simulink model "CRReferenceApplication"  (R2020a)
settings: Solver=ode23tb  StartTime=0.0  StopTime=60  FixedStep=.001  RelTol=1e-3  EnableMultiTasking=on
StartFcn:
  | %tic
StopFcn:
  | %toc
model workspace (MAT data in the model file):
  A_mu = 10
  B_reff = 8.386
  Cz = 7766.25
  DCT_Param.Transmission.Ratios = [3.78 2.18 1.43 1.03 0.935 0.84]
  DCT_Param.Transmission.Shaft_Inertia_Odd = 0.0023
  DCT_Param.Transmission.Shaft_Inertia_Even = 0.0009
  DCT_Param.Transmission.Shaft_Inertia_Output = 0.008
  DCT_Param.Transmission.Gear_Inertia = 0.001
  DCT_Param.Transmission.Gear_Efficiency = 0.94
  DCT_Param.Transmission.Gear_Ang_Vel_Thr = 0.01
  DCT_Param.Transmission.Shaft_Velocity_Odd = 0
  DCT_Param.Transmission.Shaft_Velocity_Even = 0
  DCT_Param.Transmission.Shaft_Velocity_Output = 0
  DCT_Param.Transmission.Gear_Initial_Velocity = 0
  DCT_Param.Transmission.Abstract.Compliance = 100000
  DCT_Param.Transmission.Abstract.Damping = 10000
  DCT_Param.Transmission.Abstract.Ratio_Time_Const = 0.05
  DCT_Param.Transmission.Abstract.Shift_Gear_Delay = 25
  DCT_Param.Clutch.Torque_Radius = 130
  DCT_Param.Clutch.Num_Friction_Surfaces = 4
  DCT_Param.Clutch.Engagement_Piston_Area = 0.001
  DCT_Param.Clutch.Kinetic_Friction_Coeff = 0.3
  DCT_Param.Clutch.Static_Friction_Coeff = 0.31
  DCT_Param.Clutch.Derating_Factor = 1
  DCT_Param.Clutch.Clutch_Velocity_Tolerance = 0.001
  DCT_Param.Clutch.Threshold_Pressure = 1
  DCT_Param.Clutch.Drag_Torque_Coeff = 0
  DCT_Param.Dog_Clutch.Max_Torque = 1000
  DCT_Param.Dog_Clutch.Teeth_Mean_Radius = 50
  DCT_Param.Dog_Clutch.Tooth_Height = 10
  DCT_Param.Dog_Clutch.Ring_Hub_Clearance = 3
  DCT_Param.Dog_Clutch.Ring_Stop_Stiffness = 1000000
  DCT_Param.Dog_Clutch.Ring_Stop_Damping = 1000
  DCT_Param.Dog_Clutch.Shift_Linkage_Damping = 100
  DCT_Param.Dog_Clutch.Max_Engage_Velocity = 1000000
  DCT_Param.Dog_Clutch.Tooth_Engage_Overlap = 3
  DCT_Param.Vehicle.Mass = 1600
  DCT_Param.Vehicle.Wheels_Per_Axle = 2
  DCT_Param.Vehicle.Distance_CG_FrontAxle = 1.7
  DCT_Param.Vehicle.Distance_CG_RearAxle = 2
  DCT_Param.Vehicle.Distance_CG_Ground = 0.5
  DCT_Param.Vehicle.Frontal_Area = 3
  DCT_Param.Vehicle.Aero_Drag_Coeff = 0.4
  DCT_Param.Vehicle.Initial_Velocity = 0
  DCT_Param.Vehicle.Final_Drive_Ratio = 3.7
  DCT_Param.Vehicle.Final_Drive_Efficiency = 0.86
  DCT_Param.Vehicle.Final_Drive_Vel_Thresh = 0.01
  DCT_Param.Vehicle.Side_Shaft_Inertia = 0.01
  DCT_Param.Vehicle.Side_Shaft_Initial_Velocity = 0
  DCT_Param.Vehicle.Tire.Radius = 0.312
  DCT_Param.Vehicle.Tire.Inertia = 0.5
  DCT_Param.Vehicle.Tire.Initial_Velocity = 0
  DCT_Param.Vehicle.Tire.Slip_Vel_Thresh = 0.1
  DCT_Param.Vehicle.Tire.Nominal_Vertical_Load = 4000
  DCT_Param.Vehicle.Tire.C_Coeff = 1.685
  DCT_Param.Vehicle.Tire.D_Coeff = [1.21 -0.037]
  DCT_Param.Vehicle.Tire.E_Coeff = [0.344 0.095 -0.02 0]
  DCT_Param.Vehicle.Tire.BCD_Coeff = [21.51 -0.163 0.245]
  DCT_Param.Vehicle.Tire.H_Coeff = [-0.002 0.002]
  DCT_Param.Vehicle.Tire.V_Coeff = [0 0]
  DCT_Param.ICE.Max_Power = 100000
  DCT_Param.ICE.Speed_At_Max_Power = 5500
  DCT_Param.ICE.Max_Speed = 7000
  DCT_Param.ICE.Stall_Speed = 200
  DCT_Param.ICE.Shaft_Inertia = 0.2
  DCT_Param.ICE.Initial_Velocity = 800
  DCT_Param.ICE.Idle_Ref_Spd = 800
  DCT_Param.ICE.Engine_Time_Constant = 0.2
  DCT_Param.ICE.Initial_Normalized_Throttle = 0
  DCT_Param.ICE.Speed_Threshold = 20
  DCT_Param.ICE.FC.Speed_Vector = [0 368.421052632 736.842105263 1105.26315789 1473.68421053 1842.10526316 2210.52631579 2578.94736842 2947.36842105 3315.78947368 3684.21052632 4052.63157895 4421.05263158 4789.47368421 5157.89473684 5526.31578947 5894.73684211 6263.15789474 6631.57894737 7000]
  DCT_Param.ICE.FC.Torque_Vector = [0 10.5263157895 21.0526315789 31.5789473684 42.1052631579 52.6315789474 63.1578947368 73.6842105263 84.2105263158 94.7368421053 105.263157895 115.789473684 126.315789474 136.842105263 147.368421053 157.894736842 168.421052632 178.947368421 189.473684211 200]
  DCT_Param.ICE.FC.Consumption_Table = [0.262945178015 0.225304787522 0.201465019624 0.191425874321 0.195187351614 0.212749451502 0.244112173984 0.289275519063 0.348239486736 0.421004077004 0.507569289868 0.607935125326 ... (400 elements, 20x20)]
  DCT_Param.Shift_Map_Example.Pedal_Positions = [0.1 0.4 0.5 0.9]
  DCT_Param.Shift_Map_Example.Upshift_Speeds = [11  20  26  34.5  43; 14  26  35  44.5  55; 17  31  42  52.5  65; 21  39  52  66.5  80]
  DCT_Param.Shift_Map_Example.Downshift_Speeds = [8.9  17  23.6  32.4  40.8; 11.5  22.7  32  41.6  52.2; 14  27  38.1  50  62; 18  33  48  62.6  76.2]
  DCT_Param.Shift_Map_ORIG.Pedal_Positions = [0.1 0.4 0.5 0.9]
  DCT_Param.Shift_Map_ORIG.Upshift_Speeds = [11.5  23.5  35.5  45.5  55.5; 14.5  26.5  38.5  48.5  58.5; 17.5  29.5  41.5  51.5  61.5; 20.5  32.5  44.5  54.5  64.5]
  DCT_Param.Shift_Map_ORIG.Downshift_Speeds = [8.5  20.5  32.5  42.5  52.5; 11.5  23.5  35.5  45.5  55.5; 14.5  26.5  38.5  48.5  58.5; 17.5  29.5  41.5  51.5  61.5]
  DCT_Param.Shift_Map_OPT.Pedal_Positions = [0.1 0.4 0.5 0.9]
  DCT_Param.Shift_Map_OPT.Upshift_Speeds = [17.8469  29.8469  35.8159  41.2981  46.3004; 19.2469  33.9778  43.9778  53.9778  63.9778; 24.5469  41.9778  62.1778  78.5778  106.9778; 27.5469  59.3778  99.0445  109.0445  119.0445]
  DCT_Param.Shift_Map_OPT.Downshift_Speeds = [14.8469  26.8469  32.8159  38.2981  43.3004; 16.2469  30.9778  40.9778  50.9778  60.9778; 21.5469  38.9778  59.1778  75.5778  103.9778; 24.5469  56.3778  96.0445  106.0445  116.0445]
  DCT_Param.Shift_Map.Pedal_Positions = [0.1 0.4 0.5 0.9]
  DCT_Param.Shift_Map.Upshift_Speeds = [11.5  23.5  35.5  45.5  55.5; 14.5  26.5  38.5  48.5  58.5; 17.5  29.5  41.5  51.5  61.5; 20.5  32.5  44.5  54.5  64.5]
  DCT_Param.Shift_Map.Downshift_Speeds = [8.5  20.5  32.5  42.5  52.5; 11.5  23.5  35.5  45.5  55.5; 14.5  26.5  38.5  48.5  58.5; 17.5  29.5  41.5  51.5  61.5]
  DCT_Param.Control.Clutch.Min_Lock_Pressure = 2000000
  DCT_Param.Control.Clutch.Max_Lock_Pressure = 5000000
  DCT_Param.Control.Clutch.Max_Unlock_Pressure = 500000
  DCT_Param.Control.Engine_Start_RPM = 800
  DCT_Param.Control.Engine_Stop_RPM = 790
  DCT_Param.Control.Mode_Logic_TS = 0.1
  DCT_Param.Control.ICE.Kp = 0.02
  DCT_Param.Control.ICE.Ki = 0.01
  DCT_Param.Control.Gen.Kp = 10
  DCT_Param.Control.Gen.Ki = 3
  DCT_Param.Control.Mot.Kp = 500
  DCT_Param.Control.Mot.Ki = 300
  DCT_Param.Control.Veh_Spd.Kp = 0.02
  DCT_Param.Control.Veh_Spd.Ki = 0.04
  DCT_Param.Driver.Kp = 400
  DCT_Param.Driver.Ki = 0.001
  DCT_Param.Driver.Pedal_Filter_Const = 0.01
  DCT_Param.Dog_Clutches.Pulse_Delay = 50
  DCT_Param.Dog_Clutches.Pulse_Length = 20
  DCT_Param.Animation.Teeth_Ratios = [0.338461538462 0.555555555556 0.916666666667 0.96 1.17948717949 1.92307692308]
  DCT_Param.Animation.Teeth_Ratios_Reverse = [0.458333333333 0.75]
  DCT_Param.Shift_Map_OPT506.Pedal_Positions = [0.1 0.4 0.5 0.9]
  DCT_Param.Shift_Map_OPT506.Upshift_Speeds = [18  30.2  48.3  67.3322  77.3429; 20.1  36.85  66.6178  76.7537  86.7537; 21.1  40.25  71.0189  81.0189  91.7873; 24.1  63.75  80.7523  105.9489  115.9489]
  DCT_Param.Shift_Map_OPT506.Downshift_Speeds = [15  27.2  45.3  64.3322  74.3429; 17.1  33.85  63.6178  73.7537  83.7537; 18.1  37.25  68.0189  78.0189  88.7873; 21.1  60.75  77.7523  102.9489  112.9489]
  DCT_Param.Shift_Map_OPTAbsRea176.Pedal_Positions = [0.1 0.4 0.5 0.9]
  DCT_Param.Shift_Map_OPTAbsRea176.Upshift_Speeds = [17.8469  29.8469  35.7875  44.0901  49.4243; 18.9219  34.1312  45.8256  59.7585  69.7585; 32.1719  43.4585  53.51  103.2151  114.6401; 35.1719  59.2585  99.5217  109.5217  119.5217]
  DCT_Param.Shift_Map_OPTAbsRea176.Downshift_Speeds = [14.8469  26.8469  32.7875  41.0901  46.4243; 15.9219  31.1312  42.8256  56.7585  66.7585; 29.1719  40.4585  50.51  100.2151  111.6401; 32.1719  56.2585  96.5217  106.5217  116.5217]
  DLCXref = [0 6 7 14 33.5 34 42 50 60]
  DLCYref = [0 0 -4.5 -4 -3.75 1.5 0.5 0 0]
  D_reff = 0.25826
  Downshift_Speeds = [9.5625  23.0625  36.5625  47.8125  59.0625  68.90625  78.75; 12.9375  26.4375  39.9375  51.1875  62.4375  72.84375  83.25; 16.3125  29.8125  43.3125  54.5625  65.8125  76.78125  87.75; 19.6875  33.1875  46.6875  57.9375  69.1875  80.71875  92.25]
  EngRevLim = 7000
  Pedal_Positions = [0.1 0.4 0.5 0.9]
  SUS.Stiffness = 24000
  SUS.Damping.Constant = 1262
  SUS.Damping.Rebound = [4040 4950 2883 2043]
  SUS.Damping.Compression = [3600 3420 1863 1472]
  SUS.PistonSpeed = [0.05 0.1 0.3 0.6]
  SUS.UnsprungMass.Fr = 21.0693333333
  SUS.UnsprungMass.Rr = 21.0693333333
  Upshift_Speeds = [12.9375  26.4375  39.9375  51.1875  62.4375  72.84375  83.25; 16.3125  29.8125  43.3125  54.5625  65.8125  76.78125  87.75; 19.6875  33.1875  46.6875  57.9375  69.1875  80.71875  92.25; 33  52.5  77.25  100.5  138.75  161.875  185]
  VEH.Mass = 1181
  VEH.StaticNormalFrontLoad.FR = 264.666666667
  VEH.StaticNormalFrontLoad.FL = 264.666666667
  VEH.StaticNormalRearLoad.RR = 322
  VEH.StaticNormalRearLoad.RL = 322
  VEH.WheelBase = 3.075
  VEH.FrontAxlePositionfromCG = 1.515
  VEH.RearAxlePositionfromCG = 1.504
  VEH.HeightCG = 0.134
  VEH.FrontalArea = 2.11
  VEH.DragCoefficient = 0.33
  VEH.NumberOfWheelsPerAxle = 2
  VEH.Thread.FR = 1.705
  VEH.Thread.RR = 1.705
  VEH.PitchMomentInertia = 1922.66666667
  VEH.RollMomentInertia = 432.333333333
  VEH.YawMomentInertia = 2066
  VEH.SteeringRatio = 18
  VEH.TrackWidth = 1.922
  VEH.SprungMass = 1096.72266667
  VEH.InitialLongPosition = -118
  VEH.InitialLatPosition = 3.125
  VEH.InitialVertPosition = 0
  VEH.InitialRollAngle = 0
  VEH.InitialPitchAngle = 0
  VEH.InitialYawAngle = 0
  VEH.InitialLongVel = 0
  VEH.InitialLatVel = 0
  VEH.InitialVertVel = 0
  VEH.InitialRollRate = 0
  VEH.InitialPitchRate = 0
  VEH.InitialYawRate = 0
  V_o = 16.7
  V_xlow = 1
  WH.Tire.Radius.Front = 0.384
  WH.Tire.Radius.Rear = 0.401
  WH.Tire.Sidewall = 0.245
  WH.Tire.RollingResistCoeff = 0.0103
  WH.Tire.Magic.B = 10
  WH.Tire.Magic.C = 1.9
  WH.Tire.Magic.D = 1
  WH.Tire.Magic.E = 0.97
  WH.Tire.Magic.Bx = 12
  WH.Tire.Magic.Cx = 1.9
  WH.Tire.Magic.Dx = 0.72
  WH.Tire.Magic.Ex = 0.95
  WH.Tire.Magic.By = 12
  WH.Tire.Magic.Cy = 1.3
  WH.Tire.Magic.Dy = 0.75
  WH.Tire.Magic.Ey = 0.2
  WH.Tire.Front.Ky = 40000
  WH.Tire.Rear.Ky = 40000
  WH.Tire.Kz = 320000
  WH.Tire.Damping = 100
  WH.Inertia = 1.00333333333
  WH.Mass = 11.4333333333
  WH.DampingCoefficient = 0.01
  WH.VelocityTol = 0.1
  a = 1.4
  alpha_max = 1.5
  alpha_min = -1.5
  b = 1.8
  c_zo = 209651
  epsilon = 0.1
  h = 0.134
  path.ISO3888p2.x = [0 2 12 25.5 36.5 49 61]
  path.ISO3888p2.y = [0 0 0 3.725 3.725 0 0]
  path.ISO3888p2.ylb = [1.225 1.225 1.225 4.725 4.725 1.5 1.5]
  path.ISO3888p2.yrb = [-1.225 -1.225 -1.225 2.225 2.225 -1.5 -1.5]
  path.CUSC.x = [10.668 21.336 36.576 54.864 73.152]
  path.CUSC.y = [0 0 5.1816 0 0]
  path.CUSC.ylb = [1.2192 1.2192 7.0104 1.8288 1.8288]
  path.CUSC.yrb = [-1.2192 -1.2192 3.3528 -1.8288 -1.8288]
  pio = 220000
  q_Fcx = 0
  q_Fz2 = 15.4
  q_Fzy = 0
  q_reo = 0.9974
  q_sx1 = -0.007764
  q_sx10 = 0.2824
  q_sx11 = 5.349
  q_sx12 = 0
  q_sx13 = 0
  q_sx14 = 0
  q_sx2 = 1.1915
  q_sx3 = 0.013948
  q_sx4 = 4.912
  q_sx5 = 1.02
  q_sx6 = 22.83
  q_sx7 = 0.7104
  q_sx8 = -0.023393
  q_sx9 = 0.6581
  q_sy1 = 0.00702
  q_sy2 = 0
  q_sy3 = 0.001515
  q_sy4 = 8.514e-05
  q_sy5 = 0
  q_sy6 = 0
  q_sy7 = 0.9008
  q_sy8 = -0.4089
  q_v1 = 0.0007742
  q_v2 = 0.04667
  r_Bx1 = 12.531
  r_Bx2 = 9.532
  r_Bx3 = 0
  r_By1 = 10.615
  r_By2 = 7.705
  r_By3 = 3.433e-06
  r_By4 = 0
  r_Cx1 = 1.019
  r_Cy1 = 1.0585
  r_Ex1 = -0.4487
  r_Ex2 = -0.4726
  r_Ey1 = 0.3132
  r_Ey2 = 7.63e-06
  r_Hx1 = 0.0002374
  r_Hy1 = 0.011646
  r_Hy2 = 7.63e-06
  r_Vy1 = 0.05654
  r_Vy2 = 7.63e-06
  r_Vy3 = 0
  r_Vy4 = 99.9
  r_Vy5 = 2
  r_Vy6 = 15.814
  r_o = 0.3135
  vehWidth = 2
  w = 1
undefined symbols (not defined in the file): Disabled, Right
libraries: simulink x6, autolibutils x5, vehdynlibscenariocommon x5, sim3dlib x2, vehdynlibviscommon x2, autolibshared x1, vehdynlibdriver x1, sim3dautolib x1
(part 1 of 3)
settings Model: ModifiedByFormat=The MathWorks, Inc.  SimulationMode=accelerator  OrderedModelArguments=off  Creator=The MathWorks, Inc.  LastModifiedBy=The MathWorks, Inc.
settings SolverCC: ZeroCrossAlgorithm=Adaptive  AutoInsertRateTranBlk=on  InsertRTBMode=Never (minimum delay)  DecoupledContinuousIntegration=on  MinimalZcImpactIntegration=on
settings DataIOCC: ReturnWorkspaceOutputs=off
settings DebuggingCC: SignalInfNanChecking=error  ArtificialAlgebraicLoopMsg=none  MaskedZcDiagnostic=none  IgnoredZcDiagnostic=none  ModelReferenceExtraNoncontSigs=none  PregeneratedLibrarySubsystemCodeDiagnostic=none  ArithmeticOperatorsInVariantConditions=warning
settings ModelReferenceCC: UpdateModelReferenceTargets=IfOutOfDate  ModelReferenceMinAlgLoopOccurrences=on  PropagateSignalLabelsOutOfModel=off
settings SFSimCC: SimUseLocalCustomCode=off
settings RTWCC: RTWUseLocalCustomCode=off

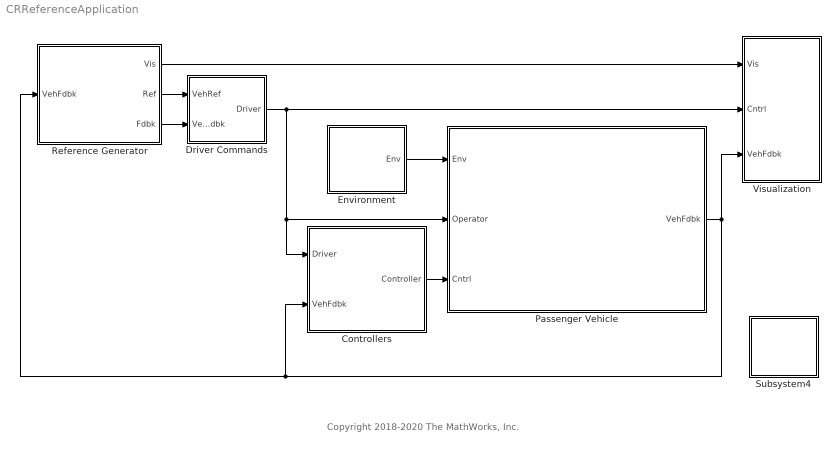
== system CRReferenceApplication ==
  note: Copyright 2018-2020 The MathWorks, Inc.
  Controllers : Subsystem
      mask Display: image('SystemControllers.png')
  Driver Commands : Subsystem  VariantControl=0  mask{driverType=Longitudinal Driver}
      mask prompts: driverType "Vehicle command mode"
      mask init:
      | [~]=vdynblksdrvrconfig(gcb)
      settings: AttributesFormatString=%<driverType>
      mask Help: eval('vdynblkshelp(''vdcrdriver'')');
      mask TypeOptions driverType: Longitudinal Driver | Predictive Driver | Open Loop
      mask Display: image('driverlatlong.png');
  Environment : Subsystem
      mask Display: disp('Environment')
  Passenger Vehicle : Subsystem
      mask Display: image('PassengerVehicle.png')
  Reference Generator : Subsystem  mask(Reference Generator){manType=Custom Maneuver, manOverride=on, prevType=Custom Maneuver, t_start=1, xdot_r=30, xdotUnit=km/h, aMode=2, omega_hw=13.5, theta_max=90, t_stop=60, ay_max=.5, ay_stop=on, XGate=174.5, xStart=2, vehW=2, lattoff=VEH.InitialLatPosition, latRefbp=DLCXref, latRef=DLCYref, t_sweep=30, theta_hw=90, theta_hw_final=.7, steerF=.7, steerA=90, tdwell=.5, steerDir=off, R=100, turnDirMask=Right, cr_ay_max=0.5, cr_ay_stop=off, SteerRef=250, simTime=60, engine3D=Disabled, SceneDesc=Straight road, dt3D=.03, defaultPos=Recommended for scene, X_o=-118, Y_o=3.125, Z_o=0, phi_o=0, theta_o=0, psi_o=0}
      mask prompts: manType "Maneuver"; manOverride "Use maneuver-specific driver, initial position, and scene"; t_start "Maneuver start time, t_start [s]:"; xdot_r "Longitudinal velocity reference, xdot_r:"; xdotUnit "Longitudinal entrance velocity setpoint units, xdotUnit []:"; omega_hw "Handwheel rate, omega_hw [deg/s]:"; theta_max "Maximum handwheel angle, theta_max [deg]:"; t_stop "Steering hold time after max angle reached, t_stop [s]:"; ay_max "Lateral acceleration threshold, ay_max [g]:"; ay_stop "Stop simulation at lateral acceleration threshold"; XGate "Inertial longitudinal position of gate entrance, XGate [m]:"; xStart "Distance after target speed to begin reference, x_start [m]:"; vehW "Vehicle width, vehW [m]:"; lattoff "Lateral offset, latoff [m]:"; latRefbp "Lateral reference position breakpoints [m]:"; latRef "Lateral reference data, latRef [m]:"; t_sweep "Swept time, t_sweep [s]:"; theta_hw "Steering amplitude, theta_hw [deg]"; theta_hw_final "Final frequency, theta_hw_final [Hz]:"; steerF "Steer frequency, steerF [Hz]:"; steerA "Steer amplitude, steerA [deg]:"; tdwell "Dwell time, tdwell [s]:"; steerDir "Change direction, steerDir"; R "Radius value, R [m]:"; turnDirMask "Turn direction"; cr_ay_max "Lateral acceleration threshold, ay_max [g]:"; cr_ay_stop "Stop simulation at lateral acceleration threshold"; SteerRef "Steering wheel angle, SteerRef [deg]:"; simTime "Simulation time, simTime [s]:"; engine3D "3D Engine"; SceneDesc "Scene:"; dt3D "Engine frame rate, dt3D [s]:"; X_o "Initial longitudinal position, X_o [m]:"; Y_o "Initial lateral position, Y_o [m]:"; Z_o "Initial vertical position, Z_o [m]:"; phi_o "Initial roll angle, phi_o [rad]:"; theta_o "Initial pitch angle, theta_o [rad]:"; psi_o "Initial yaw angle, psi_o [rad]:"
      mask help: Set parameters to configure the maneuver, driver model, and 3D environment. To set the initial vehicle position and orientation, use the parameters on the 3D Engine tab.
      mask init:
      | set_param(gcb,'prevType',get_param(gcb,'manType'))
      settings: AttributesFormatString=%<manType>
      mask Help: eval('vdynblkshelp(''vdcrrefgen'')');
      mask TypeOptions manType: Double Lane Change | Increasing Steer | Swept Sine | Sine with Dwell | Constant Radius | Custom Maneuver
      mask Callback manType:
      | [~]=vdynblksrefconfig(gcb,0);
      | [~]=vdynblksrefconfig(gcb,1);
      mask TypeOptions prevType: Double Lane Change | Increasing Steer | Swept Sine | Sine with Dwell | Constant Radius | Custom Maneuver
      mask TypeOptions xdotUnit: Reference Generator/Double Lane Change/Double Lane Change/xdotUnit | Reference Generator/Constant Radius/xdotUnit | Reference Generator/Increasing Steer/Increasing Steer/xdotUnit | Reference Generator/Sine with Dwell/Sine With Dwell/xdotUnit | Reference Generator/Swept Sine/Swept Sine/xdotUnit | Reference Generator/Custom Maneuver/Subsystem Reference/Speed Units/Unit
      mask TypeOptions omega_hw: Reference Generator/Increasing Steer/Increasing Steer/omega_hw
      mask TypeOptions theta_max: Reference Generator/Increasing Steer/Increasing Steer/theta_max
      mask TypeOptions t_stop: Reference Generator/Increasing Steer/Increasing Steer/t_stop
      mask TypeOptions ay_max: Reference Generator/Increasing Steer/Increasing Steer/ay_max
      mask TypeOptions ay_stop: Reference Generator/Increasing Steer/Increasing Steer/ay_stop
      mask Callback ay_stop:
      | if strcmp(get_param(gcb,'ay_stop'),'off')
      |     autoblksenableparameters(gcb, [], {'ay_max'},[],[],true);
      | else
      |     autoblksenableparameters(gcb,{'ay_max'},[],[],[],true);
      | end
      mask TypeOptions XGate: Reference Generator/Double Lane Change/Double Lane Change/XGate
      mask TypeOptions xStart: Reference Generator/Double Lane Change/Double Lane Change/xStart
      mask TypeOptions vehW: Reference Generator/Double Lane Change/Double Lane Change/vehW
      mask TypeOptions lattoff: Reference Generator/Double Lane Change/Double Lane Change/lattoff
      mask TypeOptions latRefbp: Reference Generator/Double Lane Change/Double Lane Change/latRefbp
      mask TypeOptions latRef: Reference Generator/Double Lane Change/Double Lane Change/latRef
      mask TypeOptions t_sweep: Reference Generator/Swept Sine/Swept Sine/t_sweep
      mask TypeOptions theta_hw: Reference Generator/Swept Sine/Swept Sine/theta_hw
      mask TypeOptions theta_hw_final: Reference Generator/Swept Sine/Swept Sine/theta_hw_final
      mask TypeOptions steerF: Reference Generator/Sine with Dwell/Sine With Dwell/steerF
      mask TypeOptions steerA: Reference Generator/Sine with Dwell/Sine With Dwell/steerA
      mask TypeOptions tdwell: Reference Generator/Sine with Dwell/Sine With Dwell/tdwell
      mask TypeOptions steerDir: Reference Generator/Sine with Dwell/Sine With Dwell/steerDir
      mask TypeOptions R: Reference Generator/Constant Radius/R
      mask TypeOptions turnDirMask: Reference Generator/Constant Radius/turnDirMask
      mask TypeOptions cr_ay_max: Reference Generator/Constant Radius/ay_max
      mask TypeOptions cr_ay_stop: Reference Generator/Constant Radius/ay_stop
      mask Callback cr_ay_stop:
      | if strcmp(get_param(gcb,'cr_ay_stop'),'off')
      |     autoblksenableparameters(gcb, [], {'cr_ay_max'},[],[],true);
      | else
      |     autoblksenableparameters(gcb,{'cr_ay_max'},[],[],[],true);
      | end
      mask TypeOptions SteerRef: Reference Generator/Custom Maneuver/Subsystem Reference/Step/After
      mask TypeOptions engine3D: 3D Engine/engine3D
      mask TypeOptions SceneDesc: 3D Engine/SceneDesc
      mask Callback SceneDesc: [~] = vdynblks3Dsceneconfig(gcb);
      mask TypeOptions dt3D: 3D Engine/dt3D
      mask TypeOptions defaultPos: Recommended for scene | User-specified
      mask TypeOptions X_o: 3D Engine/X_o
      mask TypeOptions Y_o: 3D Engine/Y_o
      mask TypeOptions Z_o: 3D Engine/Z_o
      mask TypeOptions phi_o: 3D Engine/phi_o
      mask TypeOptions theta_o: 3D Engine/theta_o
      mask TypeOptions psi_o: 3D Engine/psi_o
      mask DialogControl modTab Prompt: Model
      mask DialogControl configGroup Prompt: Configuration
      mask DialogControl ISGroup Prompt: Increasing Steer
      mask DialogControl DLCGroup Prompt: Double Lane Change
      mask DialogControl SSGroup Prompt: Swept Sine
      mask DialogControl SDGroup Prompt: Sine with Dwell
      mask DialogControl CRGroup Prompt: Constant Radius
      mask DialogControl CMGroup Prompt: Custom Maneuver
      mask DialogControl simUpdate Prompt: Set Model Simulation Time
      mask DialogControl simUpdate Callback: [~]=vdynblksrefconfig(gcb,2);
      mask DialogControl sim3DTab Prompt: 3D Engine
      mask DialogControl sim3DGroup Prompt: 3D Engine
      mask DialogControl posSetupDesc Prompt: To use these initial vehicle positions, first Apply the initial values and then click Update the model workspaces with the initial values.
      mask DialogControl setModelPos Prompt: Update model workspaces with initial values
      mask DialogControl setModelPos Callback: [~] = vdynblksmdlWSconfig(gcb);
      mask Display: image('vdbslibscen.png')
  Subsystem4 : Subsystem
      settings: OpenFcn=eval('vdynblkshelp(''vdynblksconstradius'')');
      mask Display: disp('Help')
  Visualization : Subsystem
      mask Display: disp('Visualization')
  wires:
  Passenger Vehicle/1(VehFdbk) -> Reference Generator/1("VehFdbk "), Controllers/2(VehFdbk), Visualization/3(VehFdbk)
  Controllers/1(Controller) -> Passenger Vehicle/3(Cntrl)
  Driver Commands/1(Driver) -> Passenger Vehicle/2(Operator), Controllers/1(Driver), Visualization/2(Cntrl)
  Environment/1(Env) -> Passenger Vehicle/1(Env)
  Reference Generator/1(" Vis") -> Visualization/1(Vis)
  Reference Generator/2(" Ref") -> Driver Commands/1(VehRef)
  Reference Generator/3(" Fdbk") -> Driver Commands/2(VehFdbk)

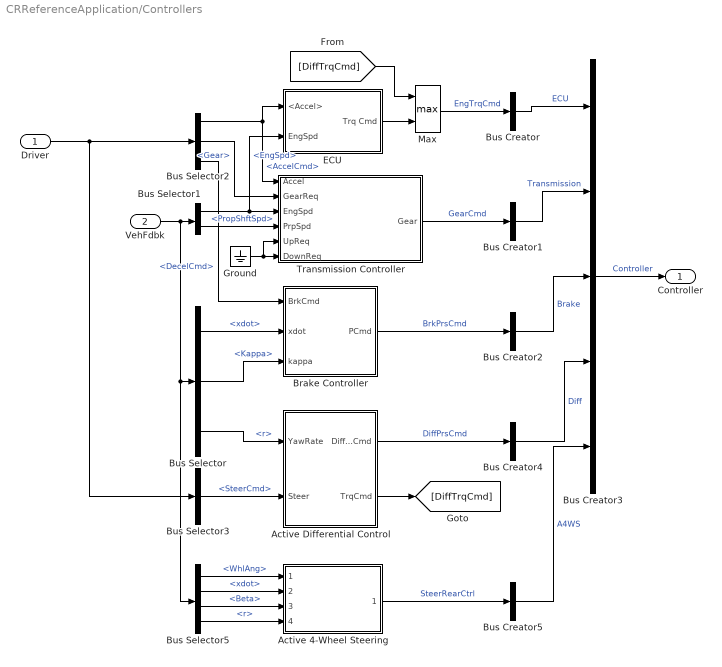
== system CRReferenceApplication/Controllers ==
  Driver : Inport
  VehFdbk : Inport  Port=2
  Active 4-Wheel Steering : Subsystem  ReferencedSubsystem=Controller
  Active Differential Control : Subsystem  Variant=on  VariantControlMode=Label  LabelModeActiveChoice=0
  Brake Controller : Subsystem
  Bus Creator{,1..2,4..5} (5 alike) : BusCreator  Inputs=1
  Bus Creator3 : BusCreator  Inputs=5
  Bus Selector : BusSelector  OutputSignals=Body.xdot,Wheels.Kappa,Body.r
  Bus Selector1 : BusSelector  OutputSignals=Driveline.EngSpd,Driveline.PropShftSpd
  Bus Selector2 : BusSelector  OutputSignals=AccelCmd,Gear,DecelCmd
  Bus Selector3 : BusSelector  OutputSignals=SteerCmd
  Bus Selector5 : BusSelector  OutputSignals=Driveline.WhlAng,Body.xdot,Body.Beta,Body.r
  ECU : Subsystem
  Ground : Ground
  Max : MinMax  Function=max  Inputs=2
  Transmission Controller : Subsystem  Variant=on  VariantControlMode=Label  VariantControl=Variant1  LabelModeActiveChoice=0
  Controller : Outport  VectorParamsAs1DForOutWhenUnconnected=off
  wires:
  Bus Selector/2 -> Brake Controller/3(kappa)  "<Kappa>"
  ECU/1(Trq Cmd) -> Max/2
  Brake Controller/1(PCmd) -> Bus Creator2/1  "BrkPrsCmd"
  VehFdbk/1 -> Bus Selector5/1, Bus Selector/1, Bus Selector1/1
  Bus Selector/1 -> Brake Controller/2(xdot)  "<xdot>"
  Driver/1 -> Bus Selector3/1, Bus Selector2/1
  Bus Selector2/1 -> ECU/1(<Accel>), Transmission Controller/1(Accel)  "<AccelCmd>"
  Bus Selector2/3 -> Brake Controller/1(BrkCmd)  "<DecelCmd>"
  Bus Creator/1 -> Bus Creator3/1  "ECU"
  Bus Creator1/1 -> Bus Creator3/2  "Transmission"
  Bus Creator2/1 -> Bus Creator3/3  "Brake"
  Bus Creator3/1 -> Controller/1  "Controller"
  Bus Creator4/1 -> Bus Creator3/4  "Diff"
  Active Differential Control/1(DiffPrsCmd) -> Bus Creator4/1  "DiffPrsCmd"
  Bus Selector3/1 -> Active Differential Control/2(Steer)  "<SteerCmd>"
  Active Differential Control/2(TrqCmd) -> [DiffTrqCmd]
  Max/1 -> Bus Creator/1  "EngTrqCmd"
  Bus Selector/3 -> Active Differential Control/1(YawRate)  "<r>"
  Bus Selector1/1 -> ECU/2(EngSpd), Transmission Controller/3(EngSpd)  "<EngSpd>"
  Bus Selector1/2 -> Transmission Controller/4(PrpSpd)  "<PropShftSpd>"
  Transmission Controller/1(" Gear") -> Bus Creator1/1  "GearCmd"
  Bus Selector2/2 -> Transmission Controller/2(GearReq)  "<Gear>"
  [DiffTrqCmd] -> Max/1
  Ground/1 -> Transmission Controller/6(DownReq), Transmission Controller/5(UpReq)
  Bus Creator5/1 -> Bus Creator3/5  "A4WS"
  Active 4-Wheel Steering/1 -> Bus Creator5/1  "SteerRearCtrl"
  Bus Selector5/1 -> Active 4-Wheel Steering/1  "<WhlAng>"
  Bus Selector5/2 -> Active 4-Wheel Steering/2  "<xdot>"
  Bus Selector5/3 -> Active 4-Wheel Steering/3  "<Beta>"
  Bus Selector5/4 -> Active 4-Wheel Steering/4  "<r>"

== system CRReferenceApplication/Driver Commands ==
  VehRef : Inport
  VehFdbk : Inport  Port=2
  AccelGround : Ground
  BrakeGround : Ground
  Driver Commands : Subsystem  Variant=on  VariantControlMode=Label  VariantControl=Variant1  LabelModeActiveChoice=0  AllowZeroVariantControls=on
  GearGround : Ground
  SteerGround : Ground
  Driver : Outport  VectorParamsAs1DForOutWhenUnconnected=off
  wires:
  VehRef/1 -> Driver Commands/1(VehRef)
  VehFdbk/1 -> Driver Commands/2(VehFdbk)
  Driver Commands/1(" Driver") -> Driver/1
  SteerGround/1 -> Driver Commands/3(SteerCmd)
  AccelGround/1 -> Driver Commands/4(Accel)
  BrakeGround/1 -> Driver Commands/5(Brake)
  GearGround/1 -> Driver Commands/6(Gear)

== system CRReferenceApplication/Environment ==
  Bus Creator1 : BusCreator  Inputs=2
  Constant3 : Constant  Value=0
  Constant4 : Constant  Value=0
  Constant5 : Constant  Value=0
  Friction : Constant  Value=ones(4,1).*1
  Ground Feedback : Subsystem  Variant=on  VariantControlMode=Label  LabelModeActiveChoice=0
  Vector Concatenate : Concatenate  NumInputs=3
  Env : Outport  VectorParamsAs1DForOutWhenUnconnected=off
  wires:
  Constant5/1 -> Vector Concatenate/3  "Z"
  Vector Concatenate/1 -> Bus Creator1/1  "Wind"
  Constant3/1 -> Vector Concatenate/1  "X"
  Constant4/1 -> Vector Concatenate/2  "Y"
  Ground Feedback/1(Ground) -> Bus Creator1/2  "Gnd"
  Bus Creator1/1 -> Env/1
  Friction/1 -> Ground Feedback/1(Friction)

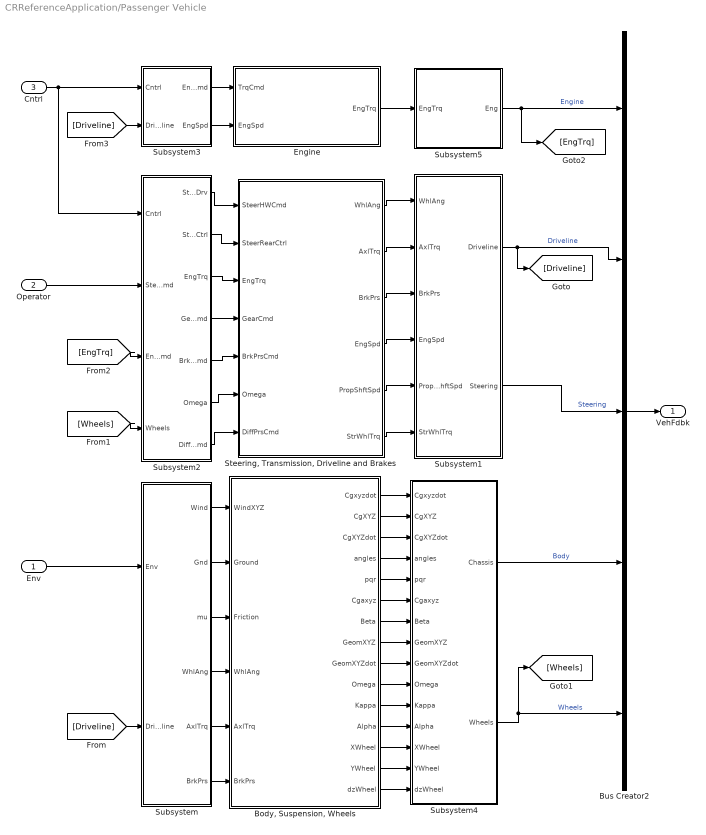
== system CRReferenceApplication/Passenger Vehicle ==
  Env : Inport
  Operator : Inport  Port=2
  Cntrl : Inport  Port=3
  "Body, Suspension, Wheels" : Subsystem  Variant=on  VariantControlMode=Label  LabelModeActiveChoice=1
  Bus Creator2 : BusCreator  Inputs=5
  Engine : Subsystem  Variant=on  VariantControlMode=Label  LabelModeActiveChoice=0
  "Steering, Transmission, Driveline and Brakes" : Subsystem  Variant=on  VariantControlMode=Label  LabelModeActiveChoice=0
  Subsystem : Subsystem
  Subsystem1 : Subsystem
  Subsystem2 : Subsystem
  Subsystem3 : Subsystem
  Subsystem4 : Subsystem
  Subsystem5 : Subsystem
  VehFdbk : Outport  VectorParamsAs1DForOutWhenUnconnected=off
  wires:
  Bus Creator2/1 -> VehFdbk/1
  Env/1 -> Subsystem/1(Env)
  Subsystem/1(Wind) -> "Body, Suspension, Wheels"/1(WindXYZ)
  Subsystem/2(Gnd) -> "Body, Suspension, Wheels"/2(Ground)
  Subsystem/3(mu) -> "Body, Suspension, Wheels"/3(Friction)
  Subsystem/4(WhlAng) -> "Body, Suspension, Wheels"/4(WhlAng)
  Subsystem/5(AxlTrq) -> "Body, Suspension, Wheels"/5(AxlTrq)
  Subsystem/6(BrkPrs) -> "Body, Suspension, Wheels"/6(BrkPrs)
  Subsystem1/1(Driveline) -> [Driveline], Bus Creator2/2  "Driveline"
  "Steering, Transmission, Driveline and Brakes"/1(WhlAng) -> Subsystem1/1(WhlAng)
  "Steering, Transmission, Driveline and Brakes"/2(AxlTrq) -> Subsystem1/2(AxlTrq)
  "Steering, Transmission, Driveline and Brakes"/3(BrkPrs) -> Subsystem1/3(BrkPrs)
  "Steering, Transmission, Driveline and Brakes"/4(EngSpd) -> Subsystem1/4(EngSpd)
  "Steering, Transmission, Driveline and Brakes"/5(PropShftSpd) -> Subsystem1/5(PropShftSpd)
  Operator/1 -> Subsystem2/2(SteerCmd)
  Cntrl/1 -> Subsystem3/1(Cntrl), Subsystem2/1(Cntrl)
  Subsystem2/1(SteerFrontDrv) -> "Steering, Transmission, Driveline and Brakes"/1(SteerHWCmd)
  Subsystem2/4(GearCmd) -> "Steering, Transmission, Driveline and Brakes"/4(GearCmd)
  Subsystem2/5(BrkPrsCmd) -> "Steering, Transmission, Driveline and Brakes"/5(BrkPrsCmd)
  Subsystem2/6(Omega) -> "Steering, Transmission, Driveline and Brakes"/6(Omega)
  Engine/1(EngTrq) -> Subsystem5/1("EngTrq ")
  Subsystem2/3(EngTrq) -> "Steering, Transmission, Driveline and Brakes"/3(EngTrq)
  Subsystem3/1(EngTrqCmd) -> Engine/1(TrqCmd)
  Subsystem3/2(EngSpd) -> Engine/2(EngSpd)
  Subsystem4/1(Chassis) -> Bus Creator2/4  "Body"
  Subsystem4/2(Wheels) -> [Wheels], Bus Creator2/5  "Wheels"
  Subsystem5/1(Eng) -> Bus Creator2/1, [EngTrq]  "Engine"
  [Driveline] -> Subsystem/2(Driveline)
  [Wheels] -> Subsystem2/4(Wheels)
  [EngTrq] -> Subsystem2/3(EngTrqCmd)
  [Driveline] -> Subsystem3/2(Driveline)
  Subsystem2/7(DiffPrsCmd) -> "Steering, Transmission, Driveline and Brakes"/7(DiffPrsCmd)
  "Steering, Transmission, Driveline and Brakes"/6(StrWhlTrq) -> Subsystem1/6(StrWhlTrq)
  Subsystem1/2(Steering) -> Bus Creator2/3  "Steering"
  "Body, Suspension, Wheels"/15(dzWheel) -> Subsystem4/15(dzWheel)
  "Body, Suspension, Wheels"/3(CgXYZdot) -> Subsystem4/3(CgXYZdot)
  "Body, Suspension, Wheels"/1(Cgxyzdot) -> Subsystem4/1(Cgxyzdot)
  "Body, Suspension, Wheels"/5(pqr) -> Subsystem4/5(pqr)
  "Body, Suspension, Wheels"/14(YWheel) -> Subsystem4/14(YWheel)
  "Body, Suspension, Wheels"/7(Beta) -> Subsystem4/7(Beta)
  "Body, Suspension, Wheels"/6(Cgaxyz) -> Subsystem4/6(Cgaxyz)
  "Body, Suspension, Wheels"/8(GeomXYZ) -> Subsystem4/8(GeomXYZ)
  "Body, Suspension, Wheels"/4(angles) -> Subsystem4/4(angles)
  "Body, Suspension, Wheels"/11(Kappa) -> Subsystem4/11(Kappa)
  "Body, Suspension, Wheels"/13(XWheel) -> Subsystem4/13(XWheel)
  "Body, Suspension, Wheels"/2(CgXYZ) -> Subsystem4/2(CgXYZ)
  "Body, Suspension, Wheels"/9(GeomXYZdot) -> Subsystem4/9(GeomXYZdot)
  "Body, Suspension, Wheels"/10(Omega) -> Subsystem4/10(Omega)
  "Body, Suspension, Wheels"/12(Alpha) -> Subsystem4/12(Alpha)
  Subsystem2/2(SteerRearCtrl) -> "Steering, Transmission, Driveline and Brakes"/2(SteerRearCtrl)

== system CRReferenceApplication/Reference Generator ==
  "VehFdbk " : Inport
  3D Engine : Subsystem  Variant=on  VariantControlMode=Label  LabelModeActiveChoice=0  mask(3D Engine){engine3D=Disabled, SceneDesc=Straight road, dt3D=dt3D, defaultPos=User-specified, X_o=X_o, Y_o=Y_o, Z_o=Z_o, phi_o=phi_o, theta_o=theta_o, psi_o=psi_o}
      mask prompts: engine3D "3D Engine"; SceneDesc "Scene:"; dt3D "Engine frame rate, dt3D [s]:"; X_o "Initial longitudinal position, X_o [m]:"; Y_o "Initial lateral position, Y_o [m]:"; Z_o "Initial vertical position, Z_o [m]:"; phi_o "Initial roll angle, phi_o [rad]:"; theta_o "Initial pitch angle, theta_o [rad]:"; psi_o "Initial yaw angle, psi_o [rad]:"
      mask help: This subsystem contains the interface blocks which permit the display of the vehicle in the 3D virtual environment. Enable it to view the simulation progress, disable it to inhibit the display.
      mask init:
      | switch get_param(gcb,'engine3D')
      |     case 'Disabled'
      |         set_param(gcb,'OverrideUsingVariant','0')
      |         try
      |             set_param([bdroot '/Environment/Ground Feedback'],'OverrideUsingVariant','0')
      |         catch
      |             disp('Warning: No ground feedback sensor not set')
      |         end
      |     case 'Enabled'
      |         set_param(gcb,'OverrideUsingVariant','1')
      |         try
      |             set_param([bdroot '/Environment/Ground Feedback'],'OverrideUsingVariant','1')
      |         catch
      |             disp('Warning: No ground feedback sensor not set')
      |         end
      |     otherwise
      |         set_param(gcb,'OverrideUsingVariant','0')
      | end
      settings: AttributesFormatString=|
      | %<SceneDesc>
      | %<engine3D>
      mask Help: eval('vdynblkshelp(''vdynblks3dengine'')');
      mask TypeOptions engine3D: Enabled | Disabled
      mask Callback engine3D:
      | switch get_param(gcb,'engine3D')
      |     case 'Disabled'
      |         set_param(gcb,'OverrideUsingVariant','0')
      |     case 'Enabled'
      |        set_param(gcb,'OverrideUsingVariant','1')
      |     otherwise
      |        set_param(gcb,'OverrideUsingVariant','0')
      | end
      mask TypeOptions SceneDesc: 3D Engine/Simulation 3D Scene Configuration/SceneDesc
      mask Callback SceneDesc: [~] = vdynblks3Dsceneconfig(gcb);
      mask TypeOptions defaultPos: Recommended for scene | User-specified
      mask DialogControl engineConfig Prompt: 3D Engine Settings
      mask DialogControl posSetup Prompt: Initial vehicle position
      mask DialogControl posSetupDesc Prompt: To use these initial vehicle positions, first Apply the initial values and then click Update the model workspaces with the initial values.
      mask DialogControl setModelPos Prompt: Update model workspaces with initial values
      mask DialogControl setModelPos Callback: [~] = vdynblksmdlWSconfig(gcb);
      mask Display: disp('3D Engine')
  Reference Generator : Subsystem  Variant=on  VariantControlMode=Label  VariantControl=Variant1  LabelModeActiveChoice=5
  " Vis" : Outport  VectorParamsAs1DForOutWhenUnconnected=off
  " Ref" : Outport  Port=2  VectorParamsAs1DForOutWhenUnconnected=off
  " Fdbk" : Outport  Port=3  VectorParamsAs1DForOutWhenUnconnected=off
  wires:
  "VehFdbk "/1 -> 3D Engine/1(VehFdbk), Reference Generator/1("VehFdbk ")
  Reference Generator/1(" Vis") -> " Vis"/1
  Reference Generator/2(" Ref") -> " Ref"/1
  Reference Generator/3(" Fdbk") -> " Fdbk"/1

== system CRReferenceApplication/Subsystem4 ==

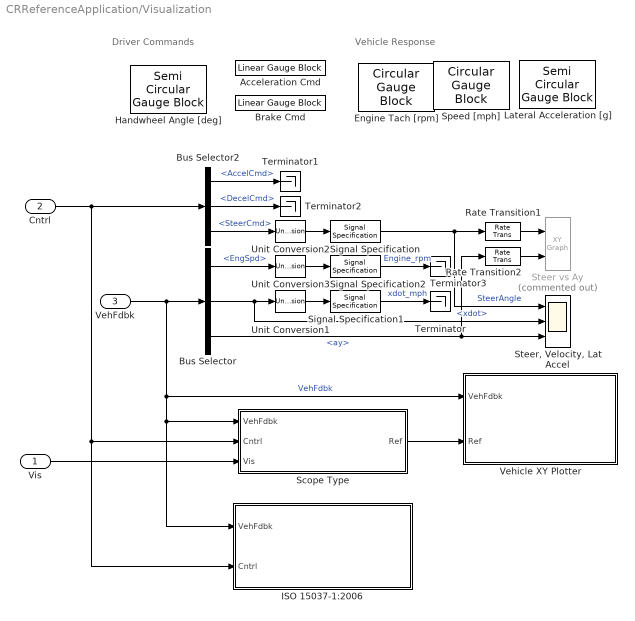
== system CRReferenceApplication/Visualization ==
  note: Vehicle Response
  note: Driver Commands
  Vis : Inport
  Cntrl : Inport  Port=2
  VehFdbk : Inport  Port=3
  Acceleration Cmd : LinearGaugeBlock  LabelPosition=Hide  ScaleMax=1  TickInterval=0.20000000000000001
  Brake Cmd : LinearGaugeBlock  LabelPosition=Hide  ScaleMax=1  TickInterval=0.20000000000000001
  Bus Selector : BusSelector  OutputSignals=Driveline.EngSpd,Body.xdot,Body.ay
  Bus Selector2 : BusSelector  OutputSignals=AccelCmd,DecelCmd,SteerCmd
  Engine Tach [rpm] : CircularGaugeBlock  LabelPosition=Hide  ScaleMax=8000  TickInterval=1000
  Handwheel Angle [deg] : SemiCircularGaugeBlock  LabelPosition=Hide  ScaleMin=-300  ScaleMax=300  TickInterval=60
  ISO 15037-1:2006 : Subsystem  StopFcn=|  Variant=on  VariantControlMode=Label  LabelModeActiveChoice=0  mask(ISO 15037-1:2006){Measurement=Disabled}
      | switch get_param(gcb,'Measurement')
      |     case 'Enabled'
      |        p=slproject.getCurrentProject;
      |        projectRoot=p.RootFolder;
      |        SySFolder=fullfile(projectRoot, 'System');
      |        Simulink.sdi.loadView([SySFolder filesep 'ISO15037_1_2006E.mldatx']);
      |        Simulink.sdi.view;
      | end
      mask prompts: Measurement "ISO Measurements"
      mask help: Enables display of ISO 15037-1:2006 standard measurement signals in the Simulation Data Inspector.
      mask init:
      | switch get_param(gcb,'Measurement')
      |     case 'Disabled'
      |         set_param(gcb,'OverrideUsingVariant','0')
      |     case 'Enabled'
      |        set_param(gcb,'OverrideUsingVariant','1')
      |     otherwise
      |        set_param(gcb,'OverrideUsingVariant','0')
      | end
      settings: AttributesFormatString=%<Measurement>
      mask Help: eval('vdynblkshelp(''iso15037'')');
      mask TypeOptions Measurement: Enabled | Disabled
      mask Callback Measurement:
      | switch get_param(gcb,'Measurement')
      |     case 'Disabled'
      |         set_param(gcb,'OverrideUsingVariant','0')
      |     case 'Enabled'
      |        set_param(gcb,'OverrideUsingVariant','1')
      |     otherwise
      |        set_param(gcb,'OverrideUsingVariant','0')
      | end
      mask Display: disp('ISO 15037-1:2006')
  Lateral Acceleration [g] : SemiCircularGaugeBlock  LabelPosition=Hide  ScaleMin=-1  ScaleMax=1  TickInterval=0.5
  Rate Transition1 : RateTransition  Deterministic=off  OutPortSampleTime=.1
  Rate Transition2 : RateTransition  Deterministic=off  OutPortSampleTime=.1
  Scope Type : Subsystem  Variant=on  VariantControlMode=Label  VariantControl=Variant1  LabelModeActiveChoice=2
  Signal Specification : SignalSpecification  Unit=deg
  Signal Specification1 : SignalSpecification  Unit=mph
  Signal Specification2 : SignalSpecification  Unit=rpm
  Speed [mph] : CircularGaugeBlock  LabelPosition=Hide  TickInterval=10
  Steer vs Ay : simulink/Sinks/XY Graph  Commented=on  xmin=-300  xmax=300  ymin=-1.5  ymax=1.5  st=.1
  "Steer, Velocity, Lat Accel" : Scope  NumInputPorts=3
  Terminator{,1..3} (4 alike) : Terminator
  Unit Conversion1 : UnitConversion
  Unit Conversion2 : UnitConversion
  Unit Conversion3 : UnitConversion
  Vehicle XY Plotter : Subsystem  Variant=on  VariantControlMode=Label  VariantControl=Variant1  LabelModeActiveChoice=1
  wires:
  Signal Specification/1 -> Rate Transition1/1, "Steer, Velocity, Lat Accel"/1  "SteerAngle"
  Bus Selector/3 -> Rate Transition2/1, "Steer, Velocity, Lat Accel"/3  "<ay>"
  Bus Selector/2 -> "Steer, Velocity, Lat Accel"/2, Unit Conversion1/1  "<xdot>"
  Unit Conversion2/1 -> Signal Specification/1
  Unit Conversion1/1 -> Signal Specification1/1
  Signal Specification1/1 -> Terminator/1  "xdot_mph"
  Bus Selector2/3 -> Unit Conversion2/1  "<SteerCmd>"
  Rate Transition1/1 -> Steer vs Ay/1
  Rate Transition2/1 -> Steer vs Ay/2
  Bus Selector2/1 -> Terminator1/1  "<AccelCmd>"
  Bus Selector2/2 -> Terminator2/1  "<DecelCmd>"
  Signal Specification2/1 -> Terminator3/1  "Engine_rpm"
  Unit Conversion3/1 -> Signal Specification2/1
  Bus Selector/1 -> Unit Conversion3/1  "<EngSpd>"
  VehFdbk/1 -> ISO 15037-1:2006/1(VehFdbk), Scope Type/1("VehFdbk "), Vehicle XY Plotter/1("VehFdbk "), Bus Selector/1  "VehFdbk"
  Cntrl/1 -> ISO 15037-1:2006/2(Cntrl), Scope Type/2(Cntrl), Bus Selector2/1
  Vis/1 -> Scope Type/3("Vis ")
  Scope Type/1(" Ref") -> Vehicle XY Plotter/2("Ref ")

== system CRReferenceApplication/Controllers/Active Differential Control ==
  note: 1) Add Subsystem or Model blocks as valid variant choices.
      | 2) You cannot connect blocks at this level. At simulation, connectivity is automatically
      | determined, based on the active variant and port name matching.
  YawRate : Inport
  Steer : Inport  Port=2
  No Control : Subsystem  VariantControl=0
  Rear Diff Controller : Subsystem  VariantControl=1
  DiffPrsCmd : Outport  VectorParamsAs1DForOutWhenUnconnected=off
  TrqCmd : Outport  Port=2  VectorParamsAs1DForOutWhenUnconnected=off

== system CRReferenceApplication/Controllers/Brake Controller ==
  BrkCmd : Inport
  xdot : Inport  Port=2
  kappa : Inport  Port=3
  Abs : Abs  ZeroCross=off
  Brake Pressure Control : Subsystem  Variant=on  VariantControlMode=Label  LabelModeActiveChoice=0
  Constant1 : Constant  Value=-20
  Gain3 : Gain
  Integrator2 : Integrator  LimitOutput=on  UpperSaturationLimit=1  LowerSaturationLimit=0
  Saturation : Saturate  UpperLimit=1  LowerLimit=0  ZeroCross=off
  Switch1 : Switch  Criteria=u2 > Threshold  Threshold=.1
  Vector Concatenate2 : Concatenate  NumInputs=4
  PCmd : Outport  VectorParamsAs1DForOutWhenUnconnected=off
  wires:
  Constant1/1 -> Switch1/3
  Gain3/1 -> Switch1/1
  Saturation/1 -> Brake Pressure Control/3(<Kappa>)  "Kappa"
  Brake Pressure Control/1(PCmd) -> PCmd/1
  kappa/1 -> Abs/1
  Integrator2/1 -> Vector Concatenate2/4, Vector Concatenate2/3, Vector Concatenate2/2, Vector Concatenate2/1
  xdot/1 -> Brake Pressure Control/2(xdot)
  Abs/1 -> Saturation/1
  Vector Concatenate2/1 -> Brake Pressure Control/1(Pref)  "Reference P"
  BrkCmd/1 -> Switch1/2, Gain3/1
  Switch1/1 -> Integrator2/1

== system CRReferenceApplication/Controllers/ECU ==
  <Accel> : Inport
  EngSpd : Inport  Port=2
  Acc to Torque Request : Gain  Gain=150
  Rev Limiter Control : Subsystem
  Signal Specification : SignalSpecification  Unit=rpm
  Unit Conversion : UnitConversion
  Trq Cmd : Outport  VectorParamsAs1DForOutWhenUnconnected=off
  wires:
  <Accel>/1 -> Acc to Torque Request/1
  Acc to Torque Request/1 -> Rev Limiter Control/1(TrqCmd)
  Rev Limiter Control/1(TrqCmdRevLimited) -> Trq Cmd/1
  EngSpd/1 -> Unit Conversion/1
  Unit Conversion/1 -> Signal Specification/1
  Signal Specification/1 -> Rev Limiter Control/2(EngSpd)  "EngSpd"

== system CRReferenceApplication/Controllers/Transmission Controller ==
  Accel : Inport
  GearReq : Inport  Port=2
  EngSpd : Inport  Port=3
  PrpSpd : Inport  Port=4
  UpReq : Inport  Port=5
  DownReq : Inport  Port=6  Unit=rad/s
  Driver - No Clutch : Subsystem  VariantControl=1
  Paddles : Subsystem  VariantControl=2
  Transmission Controller : Subsystem  VariantControl=0
  " Gear" : Outport  VectorParamsAs1DForOutWhenUnconnected=off

== system CRReferenceApplication/Driver Commands/Driver Commands ==
  VehRef : Inport
  VehFdbk : Inport  Port=2
  SteerCmd : Inport  Port=3
  Accel : Inport  Port=4
  Brake : Inport  Port=5
  Gear : Inport  Port=6
  Longitudinal Driver : Subsystem  VariantControl=0
  Open Loop Constant Radius : Subsystem  VariantControl=2
  Predictive Driver : Subsystem  VariantControl=1
  " Driver" : Outport  VectorParamsAs1DForOutWhenUnconnected=off

== system CRReferenceApplication/Environment/Ground Feedback ==
  note: 1) Add Subsystem or Model blocks as valid variant choices.
      | 2) You cannot connect blocks at this level. At simulation, connectivity is automatically
      | determined, based on the active variant and port name matching.
  Friction : Inport
  3D Engine : Subsystem  VariantControl=1
  Constant : Subsystem  VariantControl=0
  Ground : Outport  VectorParamsAs1DForOutWhenUnconnected=off

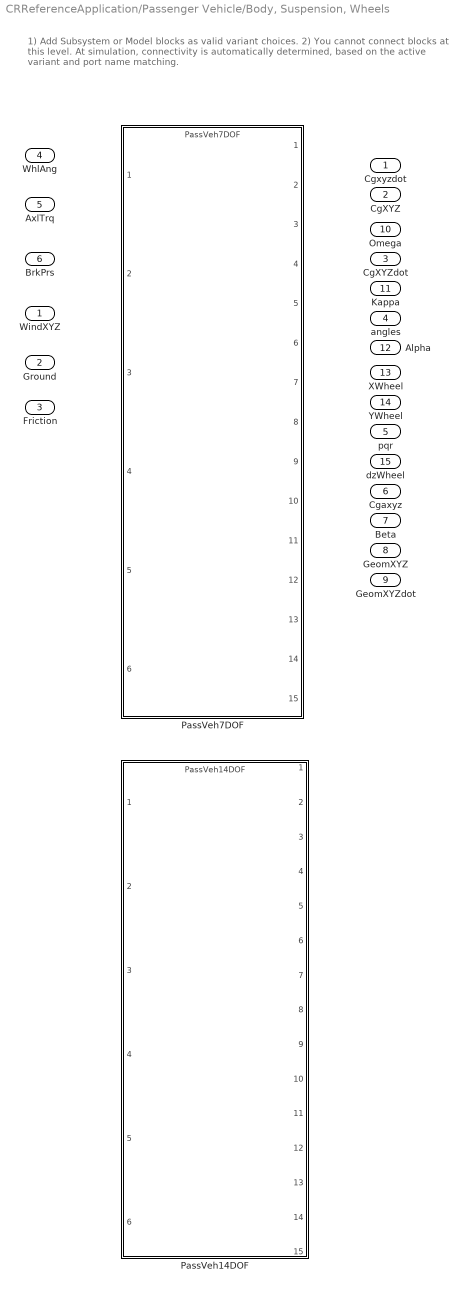
== system CRReferenceApplication/Passenger Vehicle/Body, Suspension, Wheels ==
  note: 1) Add Subsystem or Model blocks as valid variant choices.
      | 2) You cannot connect blocks at this level. At simulation, connectivity is automatically
      | determined, based on the active variant and port name matching.
  WindXYZ : Inport
  Ground : Inport  Port=2  PortDimensions=4
  Friction : Inport  Port=3  PortDimensions=4
  WhlAng : Inport  Port=4
  AxlTrq : Inport  Port=5
  BrkPrs : Inport  Port=6
  PassVeh14DOF : ModelReference  DisableCoverage=on  ModelNameDialog=PassVeh14DOF  VariantControl=3  ModelReferenceVersion=1.298
  PassVeh7DOF : ModelReference  DisableCoverage=on  ModelNameDialog=PassVeh7DOF  VariantControl=1  ModelReferenceVersion=1.153
  Cgxyzdot : Outport  VectorParamsAs1DForOutWhenUnconnected=off
  CgXYZ : Outport  Port=2  VectorParamsAs1DForOutWhenUnconnected=off
  CgXYZdot : Outport  Port=3  VectorParamsAs1DForOutWhenUnconnected=off
  angles : Outport  Port=4  VectorParamsAs1DForOutWhenUnconnected=off
  pqr : Outport  Port=5  VectorParamsAs1DForOutWhenUnconnected=off
  Cgaxyz : Outport  Port=6  VectorParamsAs1DForOutWhenUnconnected=off
  Beta : Outport  Port=7  VectorParamsAs1DForOutWhenUnconnected=off
  GeomXYZ : Outport  Port=8  VectorParamsAs1DForOutWhenUnconnected=off
  GeomXYZdot : Outport  Port=9  VectorParamsAs1DForOutWhenUnconnected=off
  Omega : Outport  Port=10  PortDimensions=4  VectorParamsAs1DForOutWhenUnconnected=off
  Kappa : Outport  Port=11  PortDimensions=4  VectorParamsAs1DForOutWhenUnconnected=off
  Alpha : Outport  Port=12  PortDimensions=4  VectorParamsAs1DForOutWhenUnconnected=off
  XWheel : Outport  Port=13  VectorParamsAs1DForOutWhenUnconnected=off
  YWheel : Outport  Port=14  VectorParamsAs1DForOutWhenUnconnected=off
  dzWheel : Outport  Port=15  VectorParamsAs1DForOutWhenUnconnected=off

== system CRReferenceApplication/Passenger Vehicle/Engine ==
  note: 1) Add Subsystem or Model blocks as valid variant choices.
      | 2) You cannot connect blocks at this level. At simulation, connectivity is automatically
      | determined, based on the active variant and port name matching.
  TrqCmd : Inport
  EngSpd : Inport  Port=2  Unit=rad/s
  Ideal Mapped Engine : ModelReference  DisableCoverage=on  ModelNameDialog=SiMappedEngineV  VariantControl=0  ModelReferenceVersion=1.324
  EngTrq : Outport  VectorParamsAs1DForOutWhenUnconnected=off

== system CRReferenceApplication/Passenger Vehicle/Steering, Transmission, Driveline and Brakes ==
  note: 1) Add Subsystem or Model blocks as valid variant choices.
      | 2) You cannot connect blocks at this level. At simulation, connectivity is automatically
      | determined, based on the active variant and port name matching.
  SteerHWCmd : Inport
  SteerRearCtrl : Inport  Port=2
  EngTrq : Inport  Port=3
  GearCmd : Inport  Port=4  OutDataTypeStr=int8
  BrkPrsCmd : Inport  Port=5  PortDimensions=4
  Omega : Inport  Port=6
  DiffPrsCmd : Inport  Port=7
  Driveline Ideal Fixed Gear : ModelReference  DisableCoverage=on  ModelNameDialog=Driveline  VariantControl=0  ModelReferenceVersion=1.220
  WhlAng : Outport  VectorParamsAs1DForOutWhenUnconnected=off
  AxlTrq : Outport  Port=2  VectorParamsAs1DForOutWhenUnconnected=off
  BrkPrs : Outport  Port=3  PortDimensions=4  VectorParamsAs1DForOutWhenUnconnected=off
  EngSpd : Outport  Port=4  Unit=rad/s  VectorParamsAs1DForOutWhenUnconnected=off
  PropShftSpd : Outport  Port=5  VectorParamsAs1DForOutWhenUnconnected=off
  StrWhlTrq : Outport  Port=6  VectorParamsAs1DForOutWhenUnconnected=off

== system CRReferenceApplication/Passenger Vehicle/Subsystem ==
  Env : Inport
  Driveline : Inport  Port=2
  Bus Selector1 : BusSelector  OutputSignals=Gnd.z.G_FL_z,Gnd.z.G_FR_z,Gnd.z.G_RL_z,Gnd.z.G_RR_z
  Bus Selector2 : BusSelector  OutputSignals=Wind
  Bus Selector3 : BusSelector  OutputSignals=Gnd.mu.mu_FL,Gnd.mu.mu_FR,Gnd.mu.mu_RL,Gnd.mu.mu_RR
  Bus Selector4 : BusSelector  OutputSignals=WhlAng,AxlTrq,BrkPrs
  Vector Concatenate : Concatenate  NumInputs=4
  Vector Concatenate1 : Concatenate  NumInputs=4
  Wind : Outport  VectorParamsAs1DForOutWhenUnconnected=off
  Gnd : Outport  Port=2  VectorParamsAs1DForOutWhenUnconnected=off
  mu : Outport  Port=3  VectorParamsAs1DForOutWhenUnconnected=off
  WhlAng : Outport  Port=4  VectorParamsAs1DForOutWhenUnconnected=off
  AxlTrq : Outport  Port=5  VectorParamsAs1DForOutWhenUnconnected=off
  BrkPrs : Outport  Port=6  VectorParamsAs1DForOutWhenUnconnected=off
  wires:
  Env/1 -> Bus Selector3/1, Bus Selector1/1, Bus Selector2/1
  Bus Selector2/1 -> Wind/1  "<Wind>"
  Bus Selector3/1 -> Vector Concatenate/1  "<mu_FL>"
  Bus Selector3/2 -> Vector Concatenate/2  "<mu_FR>"
  Bus Selector3/3 -> Vector Concatenate/3  "<mu_RL>"
  Bus Selector3/4 -> Vector Concatenate/4  "<mu_RR>"
  Vector Concatenate/1 -> mu/1
  Bus Selector1/1 -> Vector Concatenate1/1  "<G_FL_z>"
  Bus Selector1/2 -> Vector Concatenate1/2  "<G_FR_z>"
  Bus Selector1/3 -> Vector Concatenate1/3  "<G_RL_z>"
  Bus Selector1/4 -> Vector Concatenate1/4  "<G_RR_z>"
  Vector Concatenate1/1 -> Gnd/1
  Driveline/1 -> Bus Selector4/1
  Bus Selector4/2 -> AxlTrq/1  "<AxlTrq>"
  Bus Selector4/1 -> WhlAng/1  "<WhlAng>"
  Bus Selector4/3 -> BrkPrs/1  "<BrkPrs>"

== system CRReferenceApplication/Passenger Vehicle/Subsystem1 ==
  WhlAng : Inport
  AxlTrq : Inport  Port=2
  BrkPrs : Inport  Port=3
  EngSpd : Inport  Port=4
  PropShftSpd : Inport  Port=5
  StrWhlTrq : Inport  Port=6
  Bus Creator1 : BusCreator  Inputs=5
  Bus Creator2 : BusCreator  Inputs=1
  Driveline : Outport  VectorParamsAs1DForOutWhenUnconnected=off
  Steering : Outport  Port=2  VectorParamsAs1DForOutWhenUnconnected=off
  wires:
  Bus Creator1/1 -> Driveline/1  "Driveline"
  PropShftSpd/1 -> Bus Creator1/5  "PropShftSpd"
  AxlTrq/1 -> Bus Creator1/2  "AxlTrq"
  WhlAng/1 -> Bus Creator1/1  "WhlAng"
  EngSpd/1 -> Bus Creator1/4  "EngSpd"
  BrkPrs/1 -> Bus Creator1/3  "BrkPrs"
  StrWhlTrq/1 -> Bus Creator2/1  "StrWhlTrq"
  Bus Creator2/1 -> Steering/1  "Steering"

== system CRReferenceApplication/Passenger Vehicle/Subsystem2 ==
  Cntrl : Inport
  SteerCmd : Inport  Port=2
  EngTrqCmd : Inport  Port=3
  Wheels : Inport  Port=4
  Bus Selector1 : BusSelector  OutputSignals=SteerCmd
  Bus Selector2 : BusSelector  OutputSignals=Omega
  Bus Selector3 : BusSelector  OutputSignals=Transmission.GearCmd,Brake.BrkPrsCmd,Diff.DiffPrsCmd,A4WS.SteerRearCtrl
  Bus Selector4 : BusSelector  OutputSignals=EngTrq
  Data Type Conversion : DataTypeConversion
  SteerFrontDrv : Outport  VectorParamsAs1DForOutWhenUnconnected=off
  SteerRearCtrl : Outport  Port=2
  EngTrq : Outport  Port=3  VectorParamsAs1DForOutWhenUnconnected=off
  GearCmd : Outport  Port=4  VectorParamsAs1DForOutWhenUnconnected=off
  BrkPrsCmd : Outport  Port=5  VectorParamsAs1DForOutWhenUnconnected=off
  Omega : Outport  Port=6  VectorParamsAs1DForOutWhenUnconnected=off
  DiffPrsCmd : Outport  Port=7  VectorParamsAs1DForOutWhenUnconnected=off
  wires:
  Cntrl/1 -> Bus Selector3/1
  Bus Selector3/1 -> Data Type Conversion/1  "<GearCmd>"
  SteerCmd/1 -> Bus Selector1/1
  Wheels/1 -> Bus Selector2/1
  Bus Selector2/1 -> Omega/1  "<Omega>"
  Bus Selector3/2 -> BrkPrsCmd/1  "<BrkPrsCmd>"
  EngTrqCmd/1 -> Bus Selector4/1
  Bus Selector1/1 -> SteerFrontDrv/1  "<SteerCmd>"
  Bus Selector4/1 -> EngTrq/1  "<EngTrq>"
  Bus Selector3/3 -> DiffPrsCmd/1  "<DiffPrsCmd>"
  Data Type Conversion/1 -> GearCmd/1
  Bus Selector3/4 -> SteerRearCtrl/1  "<SteerRearCtrl>"

== system CRReferenceApplication/Passenger Vehicle/Subsystem3 ==
  Cntrl : Inport
  Driveline : Inport  Port=2
  Bus Selector : BusSelector  OutputSignals=ECU.EngTrqCmd
  Bus Selector1 : BusSelector  OutputSignals=EngSpd
  EngTrqCmd : Outport  VectorParamsAs1DForOutWhenUnconnected=off
  EngSpd : Outport  Port=2  VectorParamsAs1DForOutWhenUnconnected=off
  wires:
  Driveline/1 -> Bus Selector1/1
  Cntrl/1 -> Bus Selector/1
  Bus Selector/1 -> EngTrqCmd/1  "<EngTrqCmd>"
  Bus Selector1/1 -> EngSpd/1  "<EngSpd>"

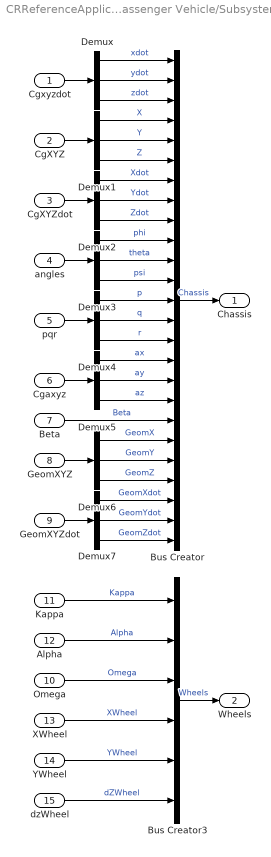
== system CRReferenceApplication/Passenger Vehicle/Subsystem4 ==
  Cgxyzdot : Inport
  CgXYZ : Inport  Port=2
  CgXYZdot : Inport  Port=3
  angles : Inport  Port=4
  pqr : Inport  Port=5
  Cgaxyz : Inport  Port=6
  Beta : Inport  Port=7
  GeomXYZ : Inport  Port=8
  GeomXYZdot : Inport  Port=9
  Omega : Inport  Port=10
  Kappa : Inport  Port=11
  Alpha : Inport  Port=12
  XWheel : Inport  Port=13
  YWheel : Inport  Port=14
  dzWheel : Inport  Port=15
  Bus Creator : BusCreator  Inputs=25
  Bus Creator3 : BusCreator  Inputs=6
  Demux{,1..7} (8 alike) : Demux  Outputs=3
  Chassis : Outport  VectorParamsAs1DForOutWhenUnconnected=off
  Wheels : Outport  Port=2  VectorParamsAs1DForOutWhenUnconnected=off
  wires:
  Bus Creator/1 -> Chassis/1  "Chassis"
  Omega/1 -> Bus Creator3/3  "Omega"
  dzWheel/1 -> Bus Creator3/6  "dZWheel"
  Kappa/1 -> Bus Creator3/1  "Kappa"
  Bus Creator3/1 -> Wheels/1  "Wheels"
  YWheel/1 -> Bus Creator3/5  "YWheel"
  XWheel/1 -> Bus Creator3/4  "XWheel"
  Alpha/1 -> Bus Creator3/2  "Alpha"
  Cgxyzdot/1 -> Demux/1
  CgXYZ/1 -> Demux1/1
  CgXYZdot/1 -> Demux2/1
  angles/1 -> Demux3/1
  pqr/1 -> Demux4/1
  Cgaxyz/1 -> Demux5/1
  GeomXYZdot/1 -> Demux7/1
  GeomXYZ/1 -> Demux6/1
  Demux/1 -> Bus Creator/1  "xdot"
  Demux/2 -> Bus Creator/2  "ydot"
  Demux/3 -> Bus Creator/3  "zdot"
  Demux1/1 -> Bus Creator/4  "X"
  Demux1/2 -> Bus Creator/5  "Y"
  Demux1/3 -> Bus Creator/6  "Z"
  Demux2/1 -> Bus Creator/7  "Xdot"
  Demux2/2 -> Bus Creator/8  "Ydot"
  Demux2/3 -> Bus Creator/9  "Zdot"
  Demux3/1 -> Bus Creator/10  "phi"
  Demux3/2 -> Bus Creator/11  "theta"
  Demux3/3 -> Bus Creator/12  "psi"
  Demux4/1 -> Bus Creator/13  "p"
  Demux4/2 -> Bus Creator/14  "q"
  Demux4/3 -> Bus Creator/15  "r"
  Demux5/1 -> Bus Creator/16  "ax"
  Demux5/2 -> Bus Creator/17  "ay"
  Demux5/3 -> Bus Creator/18  "az"
  Beta/1 -> Bus Creator/19  "Beta"
  Demux6/1 -> Bus Creator/20  "GeomX"
  Demux6/2 -> Bus Creator/21  "GeomY"
  Demux6/3 -> Bus Creator/22  "GeomZ"
  Demux7/1 -> Bus Creator/23  "GeomXdot"
  Demux7/2 -> Bus Creator/24  "GeomYdot"
  Demux7/3 -> Bus Creator/25  "GeomZdot"

== system CRReferenceApplication/Passenger Vehicle/Subsystem5 ==
  "EngTrq " : Inport
  Bus Creator : BusCreator  Inputs=1
  Eng : Outport  VectorParamsAs1DForOutWhenUnconnected=off
  wires:
  "EngTrq "/1 -> Bus Creator/1  "EngTrq"
  Bus Creator/1 -> Eng/1

== system CRReferenceApplication/Reference Generator/3D Engine ==
  note: 1) Add Subsystem or Model blocks as valid variant choices.
      | 2) You cannot connect blocks at this level. At simulation, connectivity is automatically
      | determined, based on the active variant and port name matching.
  VehFdbk : Inport
  3D Engine : Subsystem  VariantControl=1
  3D Engine Disabled : Subsystem  VariantControl=0

== system CRReferenceApplication/Reference Generator/Reference Generator ==
  "VehFdbk " : Inport
  Constant Radius : vehdynlibscenariocommon/Constant Radius  VariantControl=4  t_start=t_start  xdot_r=xdot_r  xdotUnit=km/h  R=R  turnDirMask=Right  ay_max=cr_ay_max  ay_stop=off  Parameter6=2
      settings: SourceProductBaseCode=VE
  Custom Maneuver : Subsystem  VariantControl=5
  Double Lane Change : Subsystem  VariantControl=0
  Increasing Steer : Subsystem  VariantControl=1
  Sine with Dwell : Subsystem  VariantControl=3
  Swept Sine : Subsystem  VariantControl=2
  " Vis" : Outport  VectorParamsAs1DForOutWhenUnconnected=off
  " Ref" : Outport  Port=2  VectorParamsAs1DForOutWhenUnconnected=off
  " Fdbk" : Outport  Port=3  VectorParamsAs1DForOutWhenUnconnected=off

== system CRReferenceApplication/Visualization/ISO 15037-1:2006 ==
  VehFdbk : Inport
  Cntrl : Inport  Port=2
  Disabled : Subsystem  VariantControl=0
  Enabled : Subsystem  VariantControl=1

== system CRReferenceApplication/Visualization/Scope Type ==
  "VehFdbk " : Inport
  Cntrl : Inport  Port=2
  "Vis " : Inport  Port=3
  DLC : Subsystem  VariantControl=1
  None : Subsystem  VariantControl=0
  XYZ : Subsystem  VariantControl=2
  " Ref" : Outport  VectorParamsAs1DForOutWhenUnconnected=off

== system CRReferenceApplication/Visualization/Vehicle XY Plotter ==
  "VehFdbk " : Inport
  "Ref " : Inport  Port=2
  XY View : Subsystem  VariantControl=0
  XY View Ref : Subsystem  VariantControl=1

== system CRReferenceApplication/Controllers/Active Differential Control/No Control ==
  YawRate : Inport
  Steer : Inport  Port=2
  Constant : Constant  Value=0
  Terminator : Terminator
  Terminator1 : Terminator
  Vector Concatenate2 : Concatenate  NumInputs=4
  DiffPrsCmd : Outport  VectorParamsAs1DForOutWhenUnconnected=off
  TrqCmd : Outport  Port=2  VectorParamsAs1DForOutWhenUnconnected=off
  wires:
  Constant/1 -> Vector Concatenate2/1, TrqCmd/1, Vector Concatenate2/4, Vector Concatenate2/3, Vector Concatenate2/2
  Steer/1 -> Terminator1/1
  Vector Concatenate2/1 -> DiffPrsCmd/1  "Reference P"
  YawRate/1 -> Terminator/1

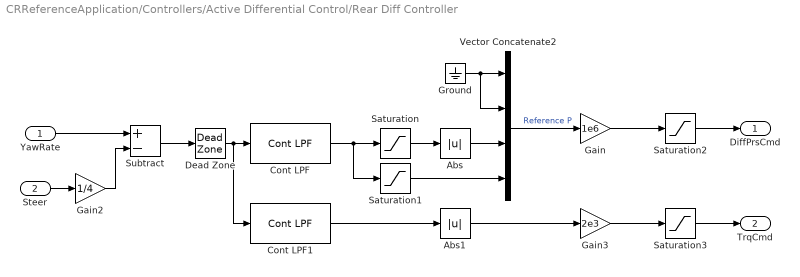
== system CRReferenceApplication/Controllers/Active Differential Control/Rear Diff Controller ==
  YawRate : Inport
  Steer : Inport  Port=2
  Abs : Abs  ZeroCross=off
  Abs1 : Abs  ZeroCross=off
  Cont LPF : autolibutils/Cont LPF  wc=10*pi  aMode=2
      settings: SourceProductBaseCode=PW,MT,VE,VP
  Cont LPF1 : autolibutils/Cont LPF  wc=1*pi  aMode=2
      settings: SourceProductBaseCode=PW,MT,VE,VP
  Dead Zone : DeadZone  LowerValue=-.01  UpperValue=.01  ZeroCross=off  SaturateOnIntegerOverflow=on
  Gain : Gain  Gain=1e6
  Gain2 : Gain  Gain=1/4
  Gain3 : Gain  Gain=2e3
  Ground : Ground
  Saturation : Saturate  UpperLimit=0  LowerLimit=-inf  ZeroCross=off
  Saturation1 : Saturate  UpperLimit=inf  LowerLimit=0  ZeroCross=off
  Saturation2 : Saturate  UpperLimit=1e7  LowerLimit=0  ZeroCross=off
  Saturation3 : Saturate  UpperLimit=200  LowerLimit=0  ZeroCross=off
  Subtract : Sum  Inputs=+-
  Vector Concatenate2 : Concatenate  NumInputs=4
  DiffPrsCmd : Outport  VectorParamsAs1DForOutWhenUnconnected=off
  TrqCmd : Outport  Port=2  VectorParamsAs1DForOutWhenUnconnected=off
  wires:
  Vector Concatenate2/1 -> Gain/1  "Reference P"
  Ground/1 -> Vector Concatenate2/2, Vector Concatenate2/1
  Steer/1 -> Gain2/1
  Saturation/1 -> Abs/1
  Saturation1/1 -> Vector Concatenate2/4
  Gain/1 -> Saturation2/1
  Abs/1 -> Vector Concatenate2/3
  Gain3/1 -> Saturation3/1
  Gain2/1 -> Subtract/2
  YawRate/1 -> Subtract/1
  Subtract/1 -> Dead Zone/1
  Abs1/1 -> Gain3/1
  Cont LPF/1 -> Saturation1/1, Saturation/1
  Saturation2/1 -> DiffPrsCmd/1
  Saturation3/1 -> TrqCmd/1
  Dead Zone/1 -> Cont LPF1/1, Cont LPF/1
  Cont LPF1/1 -> Abs1/1

== system CRReferenceApplication/Controllers/Brake Controller/Brake Pressure Control ==
  note: 1) Add Subsystem or Model blocks as valid variant choices.
      | 2) You cannot connect blocks at this level. At simulation, connectivity is automatically
      | determined, based on the active variant and port name matching.
  Pref : Inport
  xdot : Inport  Port=2
  <Kappa> : Inport  Port=3
  Bang Bang ABS : Subsystem  VariantControl=1
  Open Loop : Subsystem  VariantControl=0
  PCmd : Outport  VectorParamsAs1DForOutWhenUnconnected=off

== system CRReferenceApplication/Controllers/ECU/Rev Limiter Control ==
  TrqCmd : Inport
  EngSpd : Inport  Port=2
  1-D Lookup Table : Lookup_n-D  NumberOfTableDimensions=1  BreakpointsForDimension1=[1 1.01]  Table=[1 0]  ExtrapMethod=Clip  InternalRulePriority=Speed  RndMeth=Simplest  InputSameDT=on
  Constant : Constant  Value=EngRevLim
  Product : Product
  Product1 : Product  Inputs=*/
  TrqCmdRevLimited : Outport  VectorParamsAs1DForOutWhenUnconnected=off
  wires:
  EngSpd/1 -> Product1/1
  Product/1 -> TrqCmdRevLimited/1
  1-D Lookup Table/1 -> Product/2
  TrqCmd/1 -> Product/1
  Constant/1 -> Product1/2
  Product1/1 -> 1-D Lookup Table/1

== system CRReferenceApplication/Controllers/Transmission Controller/Driver - No Clutch ==
  GearReq : Inport
  Gear : Outport  VectorParamsAs1DForOutWhenUnconnected=off
  wires:
  GearReq/1 -> Gear/1

== system CRReferenceApplication/Controllers/Transmission Controller/Paddles ==
  Accel : Inport
  EngSpd : Inport  Port=2  Unit=rad/s
  Add1 : Sum  Inputs=+-+
  Current Gear : UnitDelay  SampleTime=-1  HasFrameUpgradeWarning=on
  Data Type Conversion2 : DataTypeConversion  OutDataTypeStr=double
  Debounce : autolibutils/Debounce  DbcOn_Cnts=10  DbcOff_Cnts=10  aMode=aMode
      settings: SourceProductBaseCode=PW,MT,VE,VP
  Debounce1 : autolibutils/Debounce  DbcOn_Cnts=10  DbcOff_Cnts=10  aMode=aMode
      settings: SourceProductBaseCode=PW,MT,VE,VP
  Demux : Demux  Outputs=2
  Detect Increase2 : simulink/Logic and Bit Operations/Detect Increase  vinit=0.0  OutDataTypeStr=boolean
  Logical Operator1 : Logic  Operator=XOR  Inputs=1  AllPortsSameDT=off  OutDataTypeStr=boolean
  Mux : Mux  Inputs=2
  Switch2 : Switch  Criteria=u2 > Threshold
  Gear : Outport  VectorParamsAs1DForOutWhenUnconnected=off
  wires:
  Debounce/1 -> Mux/1
  Mux/1 -> Detect Increase2/1
  Logical Operator1/1 -> Switch2/2
  Data Type Conversion2/1 -> Demux/1
  Demux/1 -> Add1/1
  Demux/2 -> Add1/2
  Current Gear/1 -> Add1/3, Switch2/3
  Switch2/1 -> Gear/1, Current Gear/1
  Debounce1/1 -> Mux/2
  Add1/1 -> Switch2/1
  Detect Increase2/1 -> Data Type Conversion2/1, Logical Operator1/1
  EngSpd/1 -> Debounce1/1
  Accel/1 -> Debounce/1
